simulink model "model_2"  (R2021b)
settings: Solver=VariableStepAuto  StartTime=0.0  StopTime=8  RelTol=1e-3
values from neighbouring files (symbols this model uses):
  A = [-6, 0, 0, 0; 0, 8,  0, 0; 0, 0, 2, 5; 0, 0, -5, 2]    [task_1.m]    (also in task_2.m; task_3.m = [0, 7, 0, 0; -7, 0,  0, 0; 0, 0, 0, 1; 0, 0, -1, 0]; task_4.m = [5, -9, -7, 1; -9, 5,  -1, 7; -7, -1, 5, 9; 1, 7, 9, 5])
  B = [0; 1; 9; 2]    [task_1.m]    (also in task_2.m; task_3.m = [0; 0; 0; 0]; task_4.m = [3; 3; 1; 3])
  C = [1, 0, 0, 0; 0, 1, 0, 0; 0, 0, 1, 0; 0, 0, 0, 1]    [task_1.m]    (also in task_2.m; task_3.m = [0, 5, 5, 0]; task_4.m = [2, -2, 2, 2; -2, 4, 2, 4])
  K = Y*inv(P)    [task_4.m]
  L = inv(Q)*Y1    [task_4.m]
  x0 = [10; -15; 1; -5]    [task_1.m]    (also in task_2.m; task_3.m; task_4.m)
  x_0 = [-10; 0; 0; 5]    [task_3.m]    (also in task_4.m)
settings Model: Creator=vital  LastModifiedBy=vital

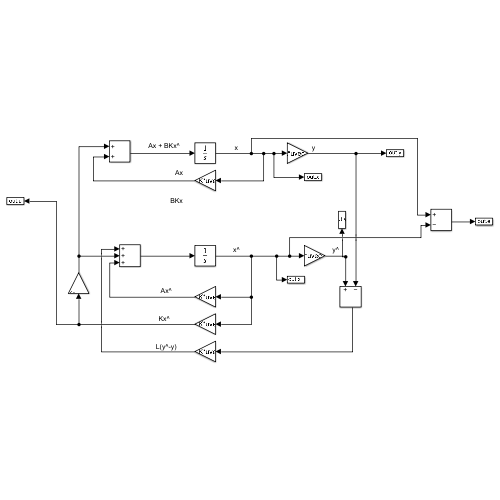
[thumbnail: Simulink's stored preview of the top-level diagram]
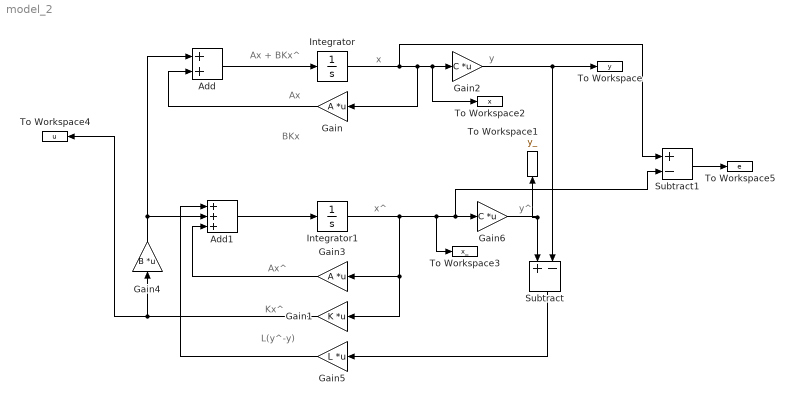
== system model_2 ==
  note: L(y^-y)
  note: Kx^
  note: Ax^
  note: y^
  note: x^
  note: y
  note: x
  note: Ax + BKx^
  note: BKx
  note: Ax
  Add : Sum
  Add1 : Sum  Inputs=+++
  Gain : Gain  Gain=A  Multiplication=Matrix(K*u) (u vector)
  Gain1 : Gain  Gain=K  Multiplication=Matrix(K*u) (u vector)
  Gain2 : Gain  Gain=C  Multiplication=Matrix(K*u) (u vector)
  Gain3 : Gain  Gain=A  Multiplication=Matrix(K*u) (u vector)
  Gain4 : Gain  Gain=B  Multiplication=Matrix(K*u) (u vector)
  Gain5 : Gain  Gain=L  Multiplication=Matrix(K*u) (u vector)
  Gain6 : Gain  Gain=C  Multiplication=Matrix(K*u) (u vector)
  Integrator : Integrator  InitialCondition=x0
  Integrator1 : Integrator  InitialCondition=x_0
  Subtract : Sum  Inputs=+-
  Subtract1 : Sum  Inputs=+-
  To Workspace : ToWorkspace  VariableName=y  SaveFormat=Timeseries  SampleTime=0.0001
  To Workspace1 : ToWorkspace  VariableName=y_  SaveFormat=Timeseries  SampleTime=-1
  To Workspace2 : ToWorkspace  VariableName=x  SaveFormat=Timeseries  SampleTime=-1
  To Workspace3 : ToWorkspace  VariableName=x_  SaveFormat=Timeseries  SampleTime=-1
  To Workspace4 : ToWorkspace  VariableName=u  SaveFormat=Timeseries  SampleTime=-1
  To Workspace5 : ToWorkspace  VariableName=e  SaveFormat=Timeseries  SampleTime=-1
  wires:
  Integrator/1 -> Subtract1/1, To Workspace2/1, Gain2/1, Gain/1
  Gain/1 -> Add/2
  Add/1 -> Integrator/1
  Gain2/1 -> Subtract/2, To Workspace/1
  Add1/1 -> Integrator1/1
  Integrator1/1 -> Gain1/1, Gain3/1, To Workspace3/1, Subtract1/2, Gain6/1
  Gain3/1 -> Add1/3
  Gain6/1 -> To Workspace1/1, Subtract/1
  Subtract/1 -> Gain5/1
  Gain5/1 -> Add1/1
  Subtract1/1 -> To Workspace5/1
  Gain1/1 -> Gain4/1, To Workspace4/1
  Gain4/1 -> Add/1, Add1/2
